simulink library "DoorRelease"  (R2022a)
settings: Solver=VariableStepAuto  StartTime=0.0  StopTime=10.0  RelTol=1e-3
settings Model: Creator=DELL  LastModifiedBy=DELL

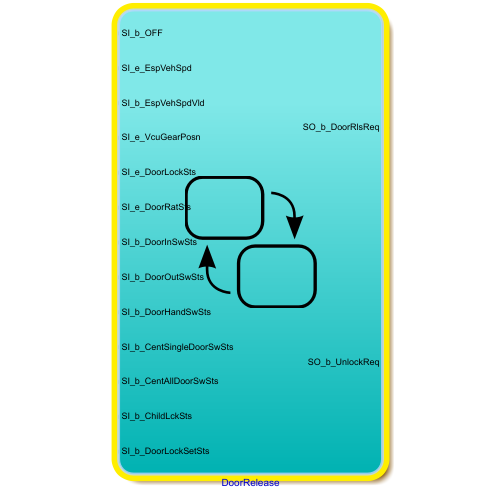
[thumbnail: Simulink's stored preview of the top-level diagram]
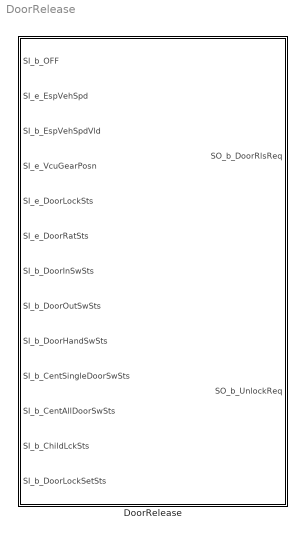
== system DoorRelease ==
  DoorRelease : Stateflow chart  TreatAsAtomicUnit=on

== stateflow chart DoorRelease/DoorRelease ==
  state DoorLockSet [parallel]
    settings: executionOrder=5
    state RlsReq [parallel]
      settings: executionOrder=1
      state Initial
        en:
        SO_b_DoorRlsReq=0;
      state TRIGGER
        state RELEASE
          en:
          SO_b_DoorRlsReq=1;
        state Wait
        (default) -> Wait
        Wait -> DoorLockSet.RlsReq.TRIGGER.RELEASE : [SI_e_DoorLockSts==1&&...
            | SI_e_DoorRatSts!=3]
      (default) -> DoorLockSet.RlsReq.Initial
      DoorLockSet.RlsReq.Initial -> DoorLockSet.RlsReq.TRIGGER : [((SI_e_EspVehSpd<=0&&SI_b_EspVehSpdVld==0)||...
          | SI_e_VcuGearPosn==1)&&...
          | SI_b_DoorLockSetSts==1&&...
          | hasChangedTo(SI_e_DoorLockSts,1)]
      DoorLockSet.RlsReq.TRIGGER -> DoorLockSet.RlsReq.Initial [order 1] : [hasChangedFrom(SI_e_VcuGearPosn,1)||...
          | (SI_e_EspVehSpd>=5&&SI_b_EspVehSpdVld==0)||...
          | (after(105,tick)&&SI_e_DoorLockSts==0)]
      DoorLockSet.RlsReq.TRIGGER -> DoorLockSet.RlsReq.Initial [order 2] : [SI_e_DoorLockSts==1&&...
          | SI_e_DoorRatSts==3]
      DoorLockSet.RlsReq.TRIGGER.RELEASE -> (junction 287) : [after(5,tick)]
      (junction 287) -> DoorLockSet.RlsReq.Initial
  state DoorIn [parallel]
    settings: executionOrder=1
    state SwValid [parallel]
      settings: executionOrder=1
      state Initial
        en:
        SL_b_DoorInSwValid=0;
      state ONCE
      state TWICE
        en:
        SL_b_DoorInSwValid=1;
      (default) -> DoorIn.SwValid.Initial
      DoorIn.SwValid.Initial -> ONCE : [hasChangedTo(SI_b_DoorInSwSts,1)&&...
          | SI_b_ChildLckSts==0]
      ONCE -> TWICE [order 1] : [hasChangedTo(SI_b_DoorInSwSts,1)&&...
          | SI_b_ChildLckSts==0]
      ONCE -> DoorIn.SwValid.Initial [order 2] : [after(200,tick)||...
          | SI_b_ChildLckSts==1]
      TWICE -> DoorIn.SwValid.Initial : [after(3,tick)]
    state RlsReq [parallel]
      settings: executionOrder=2
      state Initial
        en:
        SO_b_DoorRlsReq=0;
        SO_b_UnlockReq=0;
      state TRIGGER
        state DOOR_LOCK
          state REQ_UNLOCK
            en:
            SO_b_UnlockReq=1;
          state SUCESS_UNLOCK
          state FAIL_UNLOCK
          (default) -> DoorIn.RlsReq.TRIGGER.DOOR_LOCK.REQ_UNLOCK
          DoorIn.RlsReq.TRIGGER.DOOR_LOCK.REQ_UNLOCK -> DoorIn.RlsReq.TRIGGER.DOOR_LOCK.SUCESS_UNLOCK [order 1] : [SI_e_DoorLockSts==1]
          DoorIn.RlsReq.TRIGGER.DOOR_LOCK.REQ_UNLOCK -> DoorIn.RlsReq.TRIGGER.DOOR_LOCK.FAIL_UNLOCK [order 2] : [after(100,tick)&&...
              | SI_e_DoorLockSts==0]
        state RELEASE
          en:
          SO_b_DoorRlsReq=1;
        state DOOR_UNLOCK
        (default) -> DoorIn.RlsReq.TRIGGER.DOOR_LOCK [order 1] : [SI_e_DoorLockSts==0]
        DoorIn.RlsReq.TRIGGER.DOOR_LOCK -> DoorIn.RlsReq.TRIGGER.RELEASE : [SI_e_DoorLockSts==1&&...
            | SI_e_DoorRatSts!=3]
        DoorIn.RlsReq.TRIGGER.DOOR_UNLOCK -> DoorIn.RlsReq.TRIGGER.RELEASE : [SI_e_DoorLockSts==1&&...
            | SI_e_DoorRatSts!=3]
        (default) -> DoorIn.RlsReq.TRIGGER.DOOR_UNLOCK [order 2]
      (default) -> DoorIn.RlsReq.Initial
      DoorIn.RlsReq.Initial -> DoorIn.RlsReq.TRIGGER : [((SI_e_EspVehSpd<=0&&SI_b_EspVehSpdVld==0)||...
          | SI_e_VcuGearPosn==1)&&...
          | hasChangedTo(SL_b_DoorInSwValid,1)]
      DoorIn.RlsReq.TRIGGER -> DoorIn.RlsReq.Initial [order 1] : [hasChangedFrom(SI_e_VcuGearPosn,1)||...
          | (SI_e_EspVehSpd>=5&&SI_b_EspVehSpdVld==0)||...
          | (after(105,tick)&&SI_e_DoorLockSts==0)]
      DoorIn.RlsReq.TRIGGER -> DoorIn.RlsReq.Initial [order 2] : [SI_e_DoorLockSts==1&&...
          | SI_e_DoorRatSts==3]
      DoorIn.RlsReq.TRIGGER.RELEASE -> (junction 173) : [after(5,tick)]
      (junction 173) -> DoorIn.RlsReq.Initial
  state DoorOut [parallel]
    settings: executionOrder=3
    state SwValid [parallel]
      settings: executionOrder=1
      state Initial
        en:
        SL_b_DoorOutSwValid=SI_b_DoorOutSwSts;
        du:
        SL_b_DoorOutSwValid=SI_b_DoorOutSwSts;
      (default) -> DoorOut.SwValid.Initial
    state RlsReq [parallel]
      settings: executionOrder=2
      state Initial
        en:
        SO_b_DoorRlsReq=0;
        SO_b_UnlockReq=0;
      state TRIGGER
        state DOOR_LOCK
          state REQ_UNLOCK
            en:
            SO_b_UnlockReq=1;
          state SUCESS_UNLOCK
          state FAIL_UNLOCK
          (default) -> DoorOut.RlsReq.TRIGGER.DOOR_LOCK.REQ_UNLOCK
          DoorOut.RlsReq.TRIGGER.DOOR_LOCK.REQ_UNLOCK -> DoorOut.RlsReq.TRIGGER.DOOR_LOCK.SUCESS_UNLOCK [order 1] : [SI_e_DoorLockSts==1]
          DoorOut.RlsReq.TRIGGER.DOOR_LOCK.REQ_UNLOCK -> DoorOut.RlsReq.TRIGGER.DOOR_LOCK.FAIL_UNLOCK [order 2] : [after(100,tick)&&...
              | SI_e_DoorLockSts==0]
        state RELEASE
          en:
          SO_b_DoorRlsReq=1;
        state DOOR_UNLOCK
        (default) -> DoorOut.RlsReq.TRIGGER.DOOR_LOCK [order 1] : [SI_e_DoorLockSts==0]
        DoorOut.RlsReq.TRIGGER.DOOR_LOCK -> DoorOut.RlsReq.TRIGGER.RELEASE : [SI_e_DoorLockSts==1&&...
            | SI_e_DoorRatSts!=3]
        DoorOut.RlsReq.TRIGGER.DOOR_UNLOCK -> DoorOut.RlsReq.TRIGGER.RELEASE : [SI_e_DoorLockSts==1&&...
            | SI_e_DoorRatSts!=3]
        (default) -> DoorOut.RlsReq.TRIGGER.DOOR_UNLOCK [order 2]
      (default) -> DoorOut.RlsReq.Initial
      DoorOut.RlsReq.Initial -> DoorOut.RlsReq.TRIGGER : [((SI_e_EspVehSpd<=0&&SI_b_EspVehSpdVld==0)||...
          | SI_e_VcuGearPosn==1)&&...
          | hasChangedTo(SL_b_DoorOutSwValid,1)]
      DoorOut.RlsReq.TRIGGER -> DoorOut.RlsReq.Initial [order 1] : [hasChangedFrom(SI_e_VcuGearPosn,1)||...
          | (SI_e_EspVehSpd>=5&&SI_b_EspVehSpdVld==0)||...
          | (after(105,tick)&&SI_e_DoorLockSts==0)]
      DoorOut.RlsReq.TRIGGER -> DoorOut.RlsReq.Initial [order 2] : [SI_e_DoorLockSts==1&&...
          | SI_e_DoorRatSts==3]
      DoorOut.RlsReq.TRIGGER.RELEASE -> (junction 227) : [after(5,tick)]
      (junction 227) -> DoorOut.RlsReq.Initial
  state DoorHand [parallel]
    settings: executionOrder=4
    state SwValid [parallel]
      settings: executionOrder=2
      state Initial
        en:
        SL_b_DoorHandSwValid=0;
      state Press
      state Release
        en:
        SL_b_DoorHandSwValid=1;
      (default) -> DoorHand.SwValid.Initial
      DoorHand.SwValid.Initial -> Press : [hasChangedTo(SI_b_DoorHandSwSts,1)]
      Press -> Release [order 1] : [hasChangedTo(SI_b_DoorHandSwSts,0)]
      Press -> DoorHand.SwValid.Initial [order 2] : [after(100,tick)]
      Release -> DoorHand.SwValid.Initial : [after(3,tick)]
    state RlsReq [parallel]
      settings: executionOrder=1
      state Initial
        en:
        SO_b_DoorRlsReq=0;
        SO_b_UnlockReq=0;
      state TRIGGER
        state DOOR_LOCK
          state REQ_UNLOCK
            en:
            SO_b_UnlockReq=1;
          state SUCESS_UNLOCK
          state FAIL_UNLOCK
          (default) -> DoorHand.RlsReq.TRIGGER.DOOR_LOCK.REQ_UNLOCK
          DoorHand.RlsReq.TRIGGER.DOOR_LOCK.REQ_UNLOCK -> DoorHand.RlsReq.TRIGGER.DOOR_LOCK.SUCESS_UNLOCK [order 1] : [SI_e_DoorLockSts==1]
          DoorHand.RlsReq.TRIGGER.DOOR_LOCK.REQ_UNLOCK -> DoorHand.RlsReq.TRIGGER.DOOR_LOCK.FAIL_UNLOCK [order 2] : [after(100,tick)&&...
              | SI_e_DoorLockSts==0]
        state RELEASE
          en:
          SO_b_DoorRlsReq=1;
        state DOOR_UNLOCK
        (default) -> DoorHand.RlsReq.TRIGGER.DOOR_LOCK [order 1] : [SI_e_DoorLockSts==0]
        DoorHand.RlsReq.TRIGGER.DOOR_LOCK -> DoorHand.RlsReq.TRIGGER.RELEASE : [SI_e_DoorLockSts==1&&...
            | SI_e_DoorRatSts!=3]
        DoorHand.RlsReq.TRIGGER.DOOR_UNLOCK -> DoorHand.RlsReq.TRIGGER.RELEASE : [SI_e_DoorLockSts==1&&...
            | SI_e_DoorRatSts!=3]
        (default) -> DoorHand.RlsReq.TRIGGER.DOOR_UNLOCK [order 2]
      (default) -> DoorHand.RlsReq.Initial
      DoorHand.RlsReq.Initial -> DoorHand.RlsReq.TRIGGER : [!SI_b_OFF&&...
          | ((SI_e_EspVehSpd<=0&&SI_b_EspVehSpdVld==0)||...
          | SI_e_VcuGearPosn==1)&&...
          | hasChangedTo(SL_b_DoorHandSwValid,1)]
      DoorHand.RlsReq.TRIGGER -> DoorHand.RlsReq.Initial [order 1] : [hasChangedFrom(SI_e_VcuGearPosn,1)||...
          | (SI_e_EspVehSpd>=5&&SI_b_EspVehSpdVld==0)||...
          | (after(105,tick)&&SI_e_DoorLockSts==0)]
      DoorHand.RlsReq.TRIGGER -> DoorHand.RlsReq.Initial [order 2] : [SI_e_DoorLockSts==1&&...
          | SI_e_DoorRatSts==3]
      DoorHand.RlsReq.TRIGGER.RELEASE -> (junction 265) : [after(5,tick)]
      (junction 265) -> DoorHand.RlsReq.Initial
  state DoorCent [parallel]
    settings: executionOrder=2
    state SwValid [parallel]
      settings: executionOrder=2
      state Initial
        en:
        SL_b_CentSingleDoorSwValid=SI_b_CentSingleDoorSwSts;
        SL_b_CentAllDoorSwValid = SI_b_CentAllDoorSwSts;
        du:
        SL_b_CentSingleDoorSwValid=SI_b_CentSingleDoorSwSts;
        SL_b_CentAllDoorSwValid = SI_b_CentAllDoorSwSts;
      (default) -> DoorCent.SwValid.Initial
    state DoorCentral [parallel]
      settings: executionOrder=1
      state Initial
        en:
        SO_b_DoorRlsReq=0;
        SO_b_UnlockReq=0;
      state TRIGGER
        state DOOR_LOCK
          state REQ_UNLOCK
            en:
            SO_b_UnlockReq=1;
          state SUCESS_UNLOCK
          state FAIL_UNLOCK
          (default) -> DoorCent.DoorCentral.TRIGGER.DOOR_LOCK.REQ_UNLOCK
          DoorCent.DoorCentral.TRIGGER.DOOR_LOCK.REQ_UNLOCK -> DoorCent.DoorCentral.TRIGGER.DOOR_LOCK.SUCESS_UNLOCK [order 1] : [SI_e_DoorLockSts==1]
          DoorCent.DoorCentral.TRIGGER.DOOR_LOCK.REQ_UNLOCK -> DoorCent.DoorCentral.TRIGGER.DOOR_LOCK.FAIL_UNLOCK [order 2] : [after(100,tick)&&...
              | SI_e_DoorLockSts==0]
        state RELEASE
          en:
          SO_b_DoorRlsReq=1;
        state DOOR_UNLOCK
        (default) -> DoorCent.DoorCentral.TRIGGER.DOOR_LOCK [order 1] : [SI_e_DoorLockSts==0]
        DoorCent.DoorCentral.TRIGGER.DOOR_LOCK -> DoorCent.DoorCentral.TRIGGER.RELEASE : [SI_e_DoorLockSts==1&&...
            | SI_e_DoorRatSts!=3]
        DoorCent.DoorCentral.TRIGGER.DOOR_UNLOCK -> DoorCent.DoorCentral.TRIGGER.RELEASE : [SI_e_DoorLockSts==1&&...
            | SI_e_DoorRatSts!=3]
        (default) -> DoorCent.DoorCentral.TRIGGER.DOOR_UNLOCK [order 2]
      (default) -> DoorCent.DoorCentral.Initial
      DoorCent.DoorCentral.Initial -> DoorCent.DoorCentral.TRIGGER : [!SI_b_OFF&&...
          | ((SI_e_EspVehSpd<=0&&SI_b_EspVehSpdVld==0)||...
          | SI_e_VcuGearPosn==1)&&...
          | (hasChangedTo(SL_b_CentSingleDoorSwValid,1)||...
          | hasChangedTo(SL_b_CentAllDoorSwValid,1))]
      DoorCent.DoorCentral.TRIGGER -> DoorCent.DoorCentral.Initial [order 1] : [hasChangedFrom(SI_e_VcuGearPosn,1)||...
          | (SI_e_EspVehSpd>=5&&SI_b_EspVehSpdVld==0)||...
          | (after(105,tick)&&SI_e_DoorLockSts==0)]
      DoorCent.DoorCentral.TRIGGER -> DoorCent.DoorCentral.Initial [order 2] : [SI_e_DoorLockSts==1&&...
          | SI_e_DoorRatSts==3]
      DoorCent.DoorCentral.TRIGGER.RELEASE -> (junction 82) : [after(5,tick)]
      (junction 82) -> DoorCent.DoorCentral.Initial
  data: SI_b_OFF input boolean; SI_e_EspVehSpd input uint8; SI_b_EspVehSpdVld input boolean; SI_e_VcuGearPosn input uint8; SO_b_DoorRlsReq output boolean; SI_e_DoorLockSts input uint8; SI_e_DoorRatSts input uint8; SO_b_UnlockReq output boolean; SI_b_DoorInSwSts input boolean; SI_b_DoorOutSwSts input boolean; SI_b_DoorHandSwSts input boolean; SI_b_CentSingleDoorSwSts input boolean; SI_b_CentAllDoorSwSts input boolean; SL_b_DoorInSwValid local boolean; SL_b_CentSingleDoorSwValid local boolean; SL_b_CentAllDoorSwValid local boolean; SI_b_ChildLckSts input boolean; SL_b_DoorOutSwValid local boolean; SL_b_DoorHandSwValid local boolean; SI_b_DoorLockSetSts input boolean
